simulink model "ss_estimation_aprox_simulink"  (R2022b)
settings: Solver=VariableStepAuto  StartTime=0.0  StopTime=10.0  RelTol=1e-3
libraries: MainLibrary x1
settings Model: Creator=cotti  LastModifiedBy=cotti

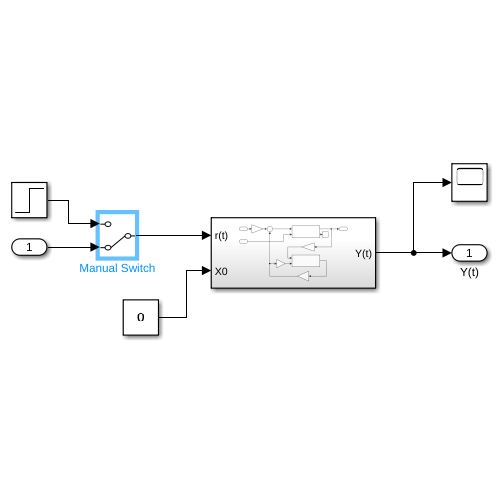
[thumbnail: Simulink's stored preview of the top-level diagram]
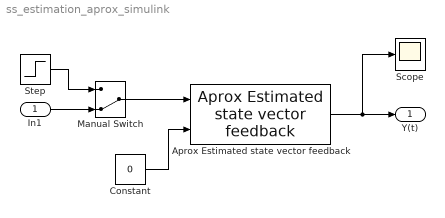
== system ss_estimation_aprox_simulink ==
  In1 : Inport
  Aprox Estimated state vector feedback : MainLibrary/Aprox Estimated state vector feedback  SystemSampleTime=-1  VariantActivationTime=update diagram  Latency=0  AutoFrameSizeCalculation=off
      settings: SourceProductName=Control Cotti
  Constant : Constant  Value=0
  Manual Switch : ManualSwitch  CurrentSetting=0
  Scope : Scope
  Step : Step  Time=0  SampleTime=0
  Y(t) : Outport
  wires:
  Constant/1 -> Aprox Estimated state vector feedback/2
  Manual Switch/1 -> Aprox Estimated state vector feedback/1
  Step/1 -> Manual Switch/1
  In1/1 -> Manual Switch/2
  Aprox Estimated state vector feedback/1 -> Scope/1, Y(t)/1
